simulink model "Discrete_Time_Integrator_verif"  (Simulink 8.4)
settings: Solver=ode45  StartTime=0.0  StopTime=10.0  RelTol=1e-3
undefined symbols (not defined in the file): DiscIntNeverNeededParam, sigbuilder_block
settings Model: Creator=Romain  LastModifiedBy=hbourbou
settings DataIOCC: SignalLoggingSaveFormat=Dataset
settings OptimizationCC: ExpressionDepthLimit=128
settings DebuggingCC: SolverPrmCheckMsg=none  FcnCallInpInsideContextMsg=EnableAllAsError  FrameProcessingCompatibilityMsg=error  StateNameClashWarn=none
settings GRTTargetCC: CombineOutputUpdateFcns=on  GRTInterface=off

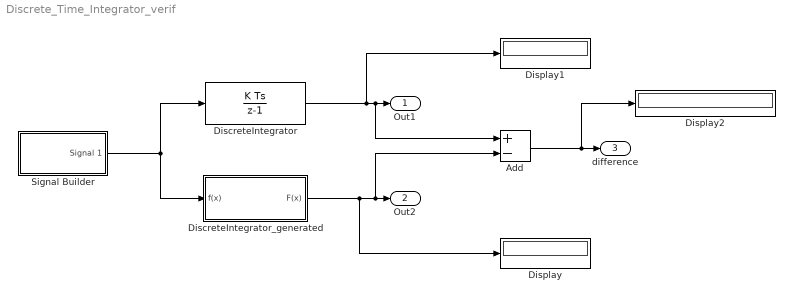
== system Discrete_Time_Integrator_verif ==
  Add : Sum  Inputs=+-
  DiscreteIntegrator : DiscreteIntegrator  InitialConditionSetting=State (most efficient)  SampleTime=-1  ICPrevOutput=DiscIntNeverNeededParam  ICPrevScaledInput=DiscIntNeverNeededParam
  DiscreteIntegrator_generated : Subsystem  TreatAsAtomicUnit=on
  Display : Display
  Display1 : Display
  Display2 : Display
  Signal Builder : Subsystem  Tag=STV Subsys  LoadFcn=sigbuilder_block('load');  StartFcn=sigbuilder_block('start');  StopFcn=sigbuilder_block('stop');  ClipboardFcn=sigbuilder_block('clipboard');  mask(Sigbuilder block){}
      mask help: Simulink:masks:SigbuilderBlock_MD
      mask init:
      | if ~strcmp(get_param(bdroot(gcbh),'SimulationStatus'),'stopped') tuvar = sigbuilder_block('maskInit'); end
      settings: CopyFcn=sigbuilder_block('copy');  DeleteFcn=sigbuilder_block('delete');  ModelCloseFcn=sigbuilder_block('modelClose');  PreSaveFcn=sigbuilder_block('preSave');  PauseFcn=sigbuilder_block('pause');  ContinueFcn=sigbuilder_block('continue');  NameChangeFcn=sigbuilder_block('namechange');  OpenFcn=sigbuilder_block('open',[437.6 199.2 550.4 400 ]);  CloseFcn=sigbuilder_block('close');
      mask Display: plot(0, 0, 100, 100,[2, 2, 32, 32, 2], [68, 8, 8, 68, 68],[32, 2], [38, 38], [32, 19, 2],[53, 60, 44], [32, 17, 17, 2],[16, 16, 31, 31]);txt = getActiveGroup(gcbh);text(2, 100, txt,'verticalAlignment', 'top');
  Out1 : Outport
  Out2 : Outport  Port=2
  difference : Outport  Port=3
  wires:
  Signal Builder/1(Signal 1) -> DiscreteIntegrator_generated/1(f(x)), DiscreteIntegrator/1
  DiscreteIntegrator/1 -> Display1/1, Add/1, Out1/1
  DiscreteIntegrator_generated/1(F(x)) -> Display/1, Add/2, Out2/1
  Add/1 -> Display2/1, difference/1

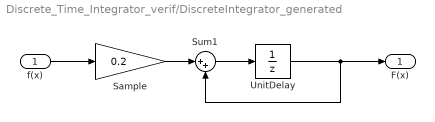
== system Discrete_Time_Integrator_verif/DiscreteIntegrator_generated ==
  f(x) : Inport
  Sample : Gain  Gain=0.2
  Sum1 : Sum  RequirementInfo={} %GIDa_8fd71d2f_119a_4852_8be5_12e2bbf92300  Inputs=|++
  UnitDelay : UnitDelay  SampleTime=0.2
  F(x) : Outport  RequirementInfo={} %GIDa_bbafc179_6ea4_4baa_a95c_c2c3921e6df7
  wires:
  f(x)/1 -> Sample/1
  UnitDelay/1 -> Sum1/2, F(x)/1
  Sum1/1 -> UnitDelay/1
  Sample/1 -> Sum1/1

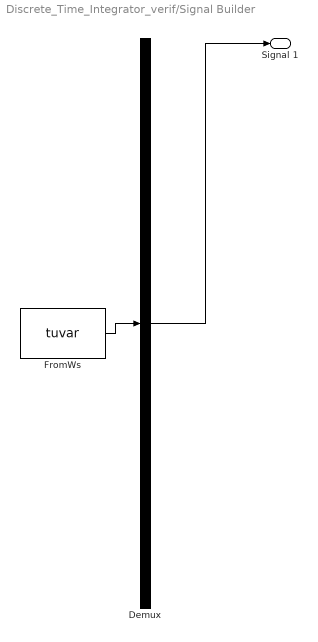
== system Discrete_Time_Integrator_verif/Signal Builder ==
  Demux : Demux  Tag=STV Demux  Outputs=1
  FromWs : FromWorkspace  Tag=STV FromWs  VariableName=tuvar  SampleTime=0  SigBuilderData=DataTag0  VnvData=DataTag1
      SigBuilderData=|
      | common.afterFinalStr = 'Extrapolate'
      | common.sampleTime = 0
      | dataSet.timeRange = [0 10]
      | dataSet.name = 'Group 1'
      | sbobj.Groups.Name = 'Group 1'
      | sbobj.Groups.Signals.Name = 'Signal 1'
      | sbobj.Groups.Signals.XData = [0 4 4 6 6 10]
      | sbobj.Groups.Signals.YData = [0 0.99 1 0.3 0.26 0]
  Signal 1 : Outport  Tag=STV Outport
  wires:
  Demux/1 -> Signal 1/1
  FromWs/1 -> Demux/1
